simulink model "augSystem"  (R2015a)
settings: Solver=ode45  StartTime=0.0  StopTime=10.0  RelTol=1e-3
values from neighbouring files (symbols this model uses):
  Arb = df(:,1:2)    [getRigidBodySS.m]
  Brb = df(:,end)    [getRigidBodySS.m]
  Crb = [Crb;zeros(1,nrb)]    [OnlyRigidBody.m]    (also in getRigidBodySS.m = dg(:,1:2))
  Drb = [Drb;zeros(1,n_inputs)]    [OnlyRigidBody.m]    (also in getRigidBodySS.m = dg(:,end))
  tau_act = 1/(2*pi*25)    (= 0.00636619772368)    [HinfSynthesis.m]
settings Model: Creator=anatole  LastModifiedBy=anatole

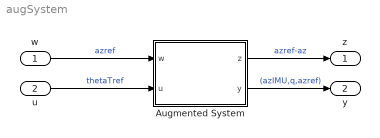
== system augSystem ==
  w : Inport
  u : Inport  Port=2
  Augmented System : Subsystem
  z : Outport
  y : Outport  Port=2
  wires:
  w/1 -> Augmented System/1(w)  "azref"
  u/1 -> Augmented System/2(u)  "thetaTref"
  Augmented System/1(z) -> z/1  "azref-az"
  Augmented System/2(y) -> y/1  "(azIMU,q,azref)"

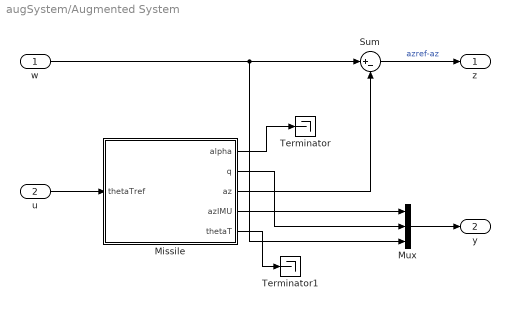
== system augSystem/Augmented System ==
  w : Inport
  u : Inport  Port=2
  Missile : Subsystem
      mask Display:
      | port_label('input', 1, '\theta_{Tref}','texmode','on')
      | 
      | port_label('output', 1, '\alpha','texmode','on')
      | port_label('output', 2, 'q','texmode','on')
      | port_label('output', 3, 'a_z','texmode','on')
      | port_label('output', 4, 'a_{zIMU}','texmode','on')
      | port_label('output', 5, '\theta_T','texmode','on')
  Mux : Mux  Inputs=3
  Sum : Sum  Inputs=|+-
  Terminator : Terminator
  Terminator1 : Terminator
  z : Outport
  y : Outport  Port=2
  wires:
  Mux/1 -> y/1
  Missile/2(q) -> Mux/2
  Missile/4(azIMU) -> Mux/1
  Missile/1(alpha) -> Terminator/1
  u/1 -> Missile/1(thetaTref)
  w/1 -> Mux/3, Sum/1
  Sum/1 -> z/1  "azref-az"
  Missile/3(az) -> Sum/2
  Missile/5("thetaT ") -> Terminator1/1

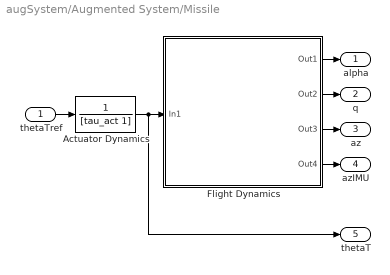
== system augSystem/Augmented System/Missile ==
  thetaTref : Inport
  Actuator Dynamics : TransferFcn  Denominator=[tau_act 1]
  Flight Dynamics : Subsystem
      mask Display:
      | port_label('input', 1, '\theta_T','texmode','on')
      | 
      | port_label('output', 1, '\alpha','texmode','on')
      | port_label('output', 2, 'q','texmode','on')
      | port_label('output', 3, 'a_z','texmode','on')
      | port_label('output', 4, 'a_{zIMU}','texmode','on')
  alpha : Outport
  q : Outport  Port=2
  az : Outport  Port=3
  azIMU : Outport  Port=4
  "thetaT " : Outport  Port=5
  wires:
  thetaTref/1 -> Actuator Dynamics/1
  Flight Dynamics/4(Out4) -> azIMU/1
  Flight Dynamics/2(Out2) -> q/1
  Flight Dynamics/1(Out1) -> alpha/1
  Actuator Dynamics/1 -> "thetaT "/1, Flight Dynamics/1(In1)
  Flight Dynamics/3(Out3) -> az/1

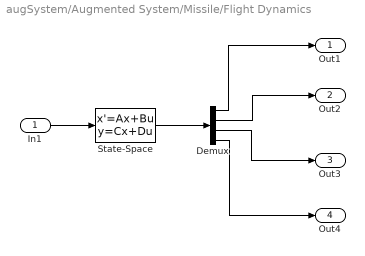
== system augSystem/Augmented System/Missile/Flight Dynamics ==
  In1 : Inport
  Demux : Demux
  State-Space : StateSpace  A=Arb  B=Brb  C=Crb  D=Drb  X0=0
  Out1 : Outport
  Out2 : Outport  Port=2
  Out3 : Outport  Port=3
  Out4 : Outport  Port=4
  wires:
  In1/1 -> State-Space/1
  State-Space/1 -> Demux/1
  Demux/3 -> Out3/1
  Demux/2 -> Out2/1
  Demux/4 -> Out4/1
  Demux/1 -> Out1/1
